simulink model "A4_model_driveline_9"  (R2024a)
settings: Solver=ode45  StartTime=0.0  StopTime=10  MaxStep=1e-3  RelTol=1e-3
values from neighbouring files (symbols this model uses):
  A = [-d_s/(J_f*r_gear^2)  d_s/(J_f*r_gear)  -c_s/(J_f*r_gear); d_s/(J_c*r_gear)  -d_s/J_c  c_s/J_c;  1/r_gear  -1  0]    [A4_41.m]
  B = [1/J_f ; 0 ; 0]    [A4_41.m]
  C_eng = [1 0 0]    [A4_41.m]
  c_s = data(5)    [A4_41.m]
  d_s = data(4)    [A4_41.m]
  J_c = data(2)    [A4_41.m]
  J_f = data(1)    [A4_41.m]
  L = P * C_eng' / inv(Rw)    [A4_41.m]
  r_gear = data(3)    [A4_41.m]
settings Model: Creator=jofr  LastModifiedBy=munav
settings SolverCC: AlgebraicLoopSolver=TrustRegion
settings DataIOCC: LimitDataPoints=on  SaveFormat=Array  SignalLoggingSaveFormat=ModelDataLogs  ReturnWorkspaceOutputs=off
settings OptimizationCC: BlockReduction=off  BooleanDataType=off  LifeSpan=inf
settings DebuggingCC: SaveWithParameterizedLinksMsg=none  UnderspecifiedInitializationDetection=Classic  MergeDetectMultiDrivingBlocksExec=none  SignalResolutionControl=TryResolveAllWithWarning  MultiTaskDSMMsg=warning  MultiTaskCondExecSysMsg=none  UnconnectedInputMsg=warning  UnconnectedOutputMsg=warning  UnconnectedLineMsg=warning  SFUnexpectedBacktrackingDiag=warning  SFNoUnconditionalDefaultTransitionDiag=warning  SFExecutionAtInitializationDiag=none  ArithmeticOperatorsInVariantConditions=warning
settings HardwareCC: ProdBitPerPointer=32  ProdBitPerSizeT=32  ProdBitPerPtrDiffT=32  ProdLargestAtomicFloat=None  ProdIntDivRoundTo=Undefined  ProdEndianess=Unspecified  ProdWordSize=32  ProdHWDeviceType=32-bit Generic  TargetUnknown=on
settings ModelReferenceCC: EnableRefExpFcnMdlSchedulingChecks=on  PropagateSignalLabelsOutOfModel=off
settings SFSimCC: SimUseLocalCustomCode=off  CustomCodeUndefinedFunction=UseInterfaceOnly
settings RTWCC: RTWUseLocalCustomCode=off  GPUComputeCapability=3.5  DLArmComputeVersion=19.05
settings CodeAppCC: StateflowObjectComments=on
settings GRTTargetCC: TargetLangStandard=C89/C90 (ANSI)
settings ConfigComp: CovMetricSettings=dw  CovSaveCumulativeToWorkspaceVar=on  CovSaveSingleToWorkspaceVar=on  CovExternalEMLEnable=off

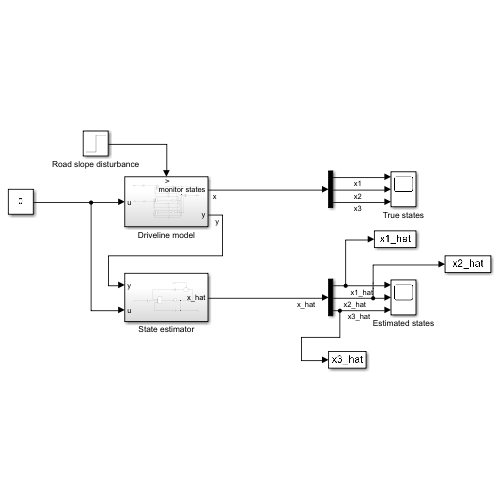
[thumbnail: Simulink's stored preview of the top-level diagram]
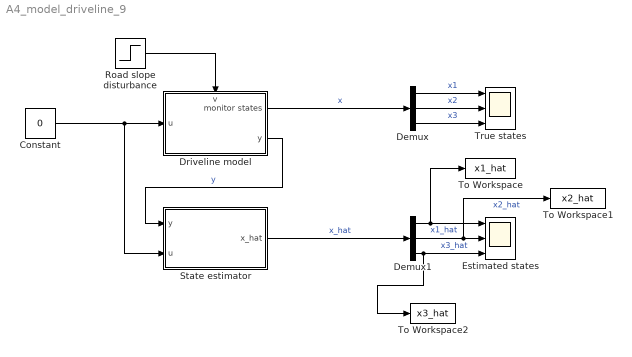
== system A4_model_driveline_9 ==
  Constant : Constant  Value=0
  Demux : Demux  Outputs=3
  Demux1 : Demux  Outputs=3
  Driveline model : Subsystem
      settings: PortSchema="{\"entries\":[{\"content\":{\"sides\":[{\"content\":{\"connectorIds\":[\"In1\"]},\"type\":\"ConnectorPlacement.EquallySpacedRectSide\",\"uuid\":\"51f5580e-5c6e-4005-9512-bdadc281ac3a\"},{\"content\":{\"connectorIds\":[\"Out1\",\"Out2\"],\"side\":\"RIGHT\"},\"type\":\"ConnectorPlacement.EquallySpacedRectSide\",\"uuid\":\"d841b77a-3407-4f39-8145-3c049402f25c\"},{\"content\":{\"connectorIds\":[\"In2\"],\"side\":\"TOP\"},\"type\":\"ConnectorPlacement.EquallySpacedRectSide\",\"uuid\":\"59296623-80a5-431d-9ae6-ee17199b70f7\"},{\"content\":{\"connectorIds\":[],\"side\":\"HIDDEN\"},\"type\":\"ConnectorPlacement.EquallySpacedRectSide\",\"uuid\":\"7f9b0e8e-917b-4707-8477-31ec1d3d2eee\"}]},\"type\":\"ConnectorPlacement.EquallySpacedConnector\",\"uuid\":\"993d3ed7-592f-4af3-96ae-7f032c513b4f\"}],\"packageUris\":[\"http://schema.mathworks.com/mf0/Connector/R2020b\"],\"version\":\"1.0\"}"
  Estimated states : Scope  NumInputPorts=3
  Road slope disturbance : Step  Time=30  After=0.1  SampleTime=0
  State estimator : Subsystem
  To Workspace : ToWorkspace  VariableName=x1_hat  SaveFormat=Timeseries  SampleTime=-1
  To Workspace1 : ToWorkspace  VariableName=x2_hat  SaveFormat=Timeseries  SampleTime=-1
  To Workspace2 : ToWorkspace  VariableName=x3_hat  SaveFormat=Timeseries  SampleTime=-1
  True states : Scope  NumInputPorts=3
  wires:
  Road slope disturbance/1 -> Driveline model/2(v)
  Driveline model/2(y) -> State estimator/1(y)  "y"
  Driveline model/1(monitor states) -> Demux/1  "x"
  Demux/3 -> True states/3  "x3"
  Demux/1 -> True states/1  "x1"
  Demux/2 -> True states/2  "x2"
  Demux1/2 -> To Workspace1/1, Estimated states/2  "x2_hat"
  Demux1/1 -> To Workspace/1, Estimated states/1  "x1_hat"
  Demux1/3 -> To Workspace2/1, Estimated states/3  "x3_hat"
  State estimator/1(x_hat) -> Demux1/1  "x_hat"
  Constant/1 -> State estimator/2(u), Driveline model/1(u)

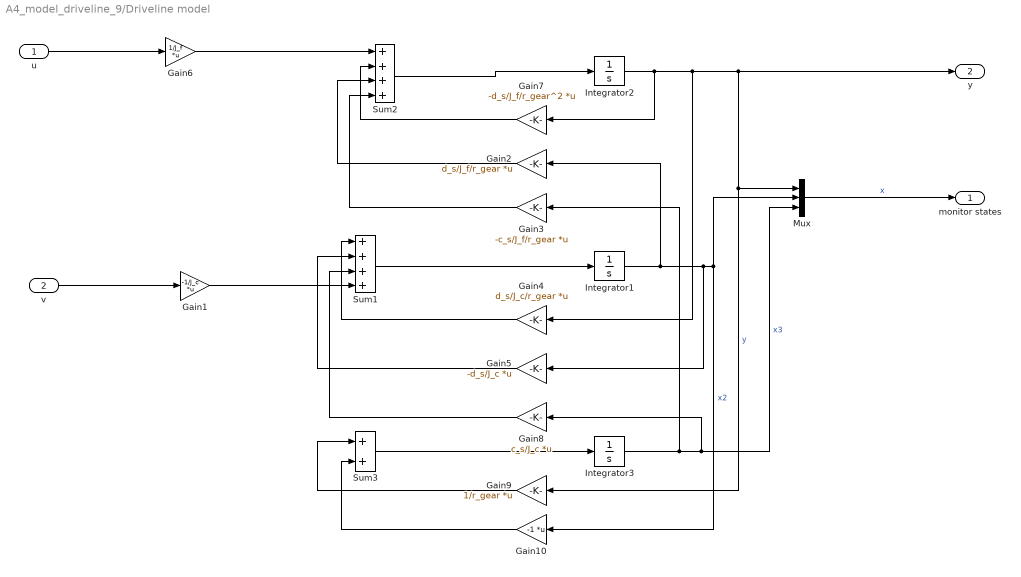
== system A4_model_driveline_9/Driveline model ==
  u : Inport
  v : Inport  Port=2
  Gain1 : Gain  Gain=-1/J_c  Multiplication=Matrix(K*u)
  Gain10 : Gain  Gain=-1  Multiplication=Matrix(K*u)
  Gain2 : Gain  Gain=d_s/J_f/r_gear  Multiplication=Matrix(K*u)
  Gain3 : Gain  Gain=-c_s/J_f/r_gear  Multiplication=Matrix(K*u)
  Gain4 : Gain  Gain=d_s/J_c/r_gear  Multiplication=Matrix(K*u)
  Gain5 : Gain  Gain=-d_s/J_c  Multiplication=Matrix(K*u)
  Gain6 : Gain  Gain=1/J_f  Multiplication=Matrix(K*u)
  Gain7 : Gain  Gain=-d_s/J_f/r_gear^2  Multiplication=Matrix(K*u)
  Gain8 : Gain  Gain=c_s/J_c  Multiplication=Matrix(K*u)
  Gain9 : Gain  Gain=1/r_gear  Multiplication=Matrix(K*u)
  Integrator1 : Integrator  InitialCondition=120/r_gear
  Integrator2 : Integrator  InitialCondition=120
  Integrator3 : Integrator
  Mux : Mux  Inputs=3
  Sum1 : Sum  Inputs=++++
  Sum2 : Sum  Inputs=++++
  Sum3 : Sum
  monitor states : Outport
  y : Outport  Port=2
  wires:
  Integrator2/1 -> Gain4/1, y/1, Mux/1, Gain9/1, Gain7/1  "y"
  Sum2/1 -> Integrator2/1
  Gain6/1 -> Sum2/1
  u/1 -> Gain6/1
  Gain7/1 -> Sum2/2
  v/1 -> Gain1/1
  Integrator1/1 -> Gain2/1, Gain5/1, Gain10/1, Mux/2  "x2"
  Integrator3/1 -> Gain3/1, Gain8/1, Mux/3  "x3"
  Gain2/1 -> Sum2/3
  Gain3/1 -> Sum2/4
  Sum1/1 -> Integrator1/1
  Gain4/1 -> Sum1/1
  Gain5/1 -> Sum1/2
  Gain8/1 -> Sum1/3
  Gain1/1 -> Sum1/4
  Sum3/1 -> Integrator3/1
  Gain10/1 -> Sum3/2
  Gain9/1 -> Sum3/1
  Mux/1 -> monitor states/1  "x"

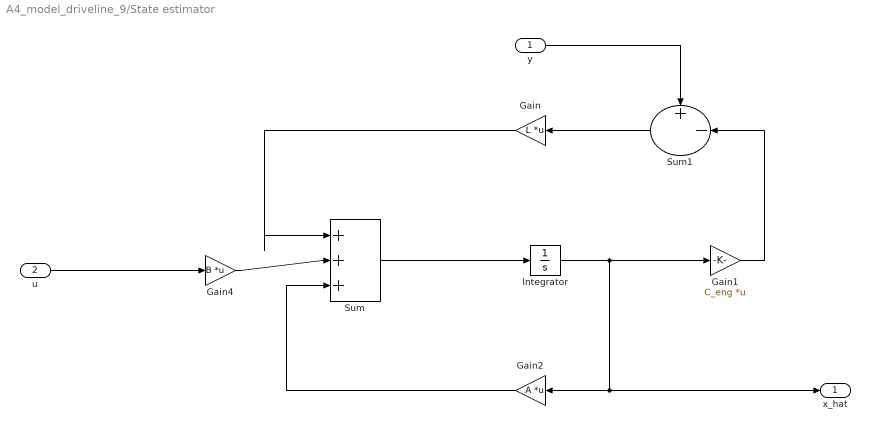
== system A4_model_driveline_9/State estimator ==
  y : Inport
  u : Inport  Port=2
  Gain : Gain  Gain=L  Multiplication=Matrix(K*u)
  Gain1 : Gain  Gain=C_eng  Multiplication=Matrix(K*u)
  Gain2 : Gain  Gain=A  Multiplication=Matrix(K*u)
  Gain4 : Gain  Gain=B  Multiplication=Matrix(K*u)
  Integrator : Integrator  InitialCondition="[0  0  -0.1]'"
  Sum : Sum  Inputs=|+++
  Sum1 : Sum  Inputs=+-|
  x_hat : Outport
  wires:
  Sum/1 -> Integrator/1
  u/1 -> Gain4/1
  Gain/1 -> Sum/1
  y/1 -> Sum1/1
  Integrator/1 -> x_hat/1, Gain2/1, Gain1/1
  Gain2/1 -> Sum/3
  Gain4/1 -> Sum/2
  Sum1/1 -> Gain/1
  Gain1/1 -> Sum1/2
